simulink model "rtwdemo_reusable"  (Simulink 6.0)
settings: Solver=FixedStepDiscrete  StartTime=0.0  StopTime=10.0  RelTol=1e-3
PostLoadFcn:
  | rtwdemo_reusable_data
values from neighbouring files (symbols this model uses):
  k1 = Simulink.Parameter    [rtwdemo_reusable_data.m]
libraries: rtwdemowidgets x2
settings Model: Creator=The MathWorks Inc.  LastModifiedBy=batserve  ExtModeArmWhenConnect=off  ExtModeAutoUpdateStatusClock=off
settings DataIOCC: SaveOutput=off  SaveTime=off  SignalLoggingName=sigsOut
settings OptimizationCC: InlineParams=on  EnforceIntegerDowncast=off  StateBitsets=on  DataBitsets=on  UseTempVars=on  ZeroExternalMemoryAtStartup=off  ZeroInternalMemoryAtStartup=off  InitFltsAndDblsToZero=off  NoFixptDivByZeroProtection=on  OptimizeModelRefInitCode=on  LifeSpan=1
settings DebuggingCC: CheckExecutionContextPreStartOutputMsg=on  CheckExecutionContextRuntimeOutputMsg=on  SolverPrmCheckMsg=none  UnconnectedInputMsg=none  UnconnectedOutputMsg=none  UnconnectedLineMsg=none
settings RTWCC: SystemTargetFile=ert.tlc  TLCOptions=-p0 -aWarnNonSaturatedBlocks=0  TemplateMakefile=ert_default_tmf  GenerateReport=on  RTWVerbose=off  ProcessScript=ert_make_rtw_hook  IncludeHyperlinkInReport=on  LaunchReport=on
settings CodeAppCC: ForceParamTrailComments=on  IgnoreCustomStorageClasses=off  SimulinkDataObjDesc=on  PrefixModelToSubsysFcnNames=off  CustomSymbolStr=$N$M  InsertBlockDesc=on
settings ERTTargetCC: TargetFcnLib=ansi_tfl_tmw.mat  GenFloatMathFcnCalls=ANSI_C  GenerateSampleERTMain=on  IncludeMdlTerminateFcn=off  MultiInstanceERTCode=on  SupportNonFinite=off  SupportContinuousTime=on  SupportNonInlinedSFcns=on  InlinedParameterPlacement=NonHierarchical  RootIOFormat=Structure Reference  ERTCustomFileTemplate=example_file_process.tlc  InitialValueSource=Model

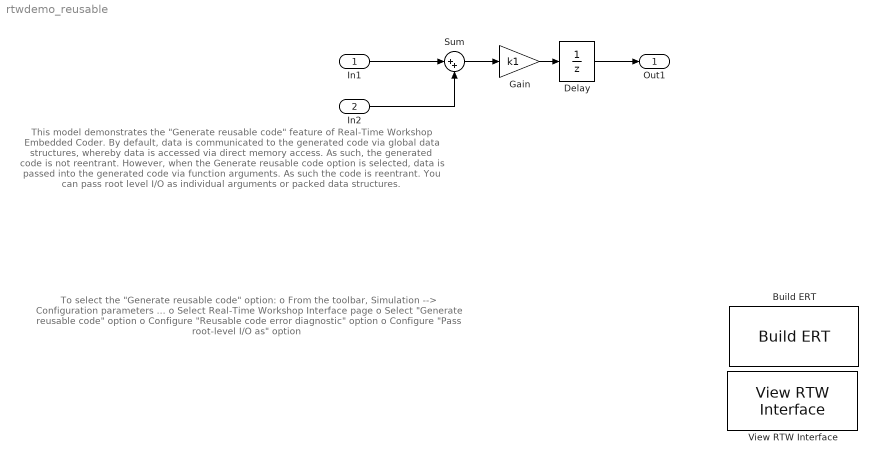
== system rtwdemo_reusable ==
  note: This model demonstrates the "Generate reusable code" feature of Real-Time Workshop Embedded Coder.
      |
      | By default, data is communicated to the generated code via global data structures, whereby data
      | is accessed via direct memory access.  As such, the generated code is not reentrant.  However,
      | when the Generate reusable code option is selected, data is passed into the generated code via
      | function arguments.  As such the code is reentrant.
      |
      | You can pass root level I/O as individual arguments or packed data structures.
  note: To select the "Generate reusable code" option:
      |
      | o From the toolbar, Simulation --> Configuration parameters ...
      | o Select Real-Time Workshop Interface page
      | o Select "Generate reusable code" option
      | o Configure "Reusable code error diagnostic" option
      | o Configure "Pass root-level I/O as" option
  In1 : Inport  Port=1  SampleTime=1  LatchInput=off
  In2 : Inport  Port=2  SampleTime=1  LatchInput=off
  Build ERT : rtwdemowidgets/Build ERT  attrib_overrides={'MultiInstanceERTCode', 'RootIOFormat'}
  Delay : UnitDelay
  Gain : Gain  Gain=k1  SaturateOnIntegerOverflow=on
  Sum : Sum  Inputs=|++  SaturateOnIntegerOverflow=on  InputSameDT=on
  View RTW Interface : rtwdemowidgets/View RTW Interface
  Out1 : Outport
  wires:
  In1/1 -> Sum/1
  Sum/1 -> Gain/1
  In2/1 -> Sum/2
  Gain/1 -> Delay/1
  Delay/1 -> Out1/1
